simulink model "mu_estimate"  (R2021b)
settings: Solver=ode4  StartTime=0.0  StopTime=5  FixedStep=0.001  RelTol=1e-3
values from neighbouring files (symbols this model uses):
  afx_f = [1.736519934348130,-2.903281841026900e-04,2.651682004580759,7.000047010028531e+04,3.270011055825476e+03,-0.001252141095807,1.596836353939939]    [VehicleParamsFEM20.m]    (also in VehicleParamsFEM20_Gear17.m; VehicleParamsFEM21.m)
  agx_f = [0.230000000000000,2.936116597489246e+04,7.137436879966481e+03,0,0]    [VehicleParamsFEM20.m]    (also in VehicleParamsFEM20_Gear17.m; VehicleParamsFEM21.m)
  Cd = Cd/(40/3.6)^2    (= 0.6885)    [VehicleParamsFEM20.m]    (also in VehicleParamsFEM20_Gear17.m; VehicleParamsFEM21.m)
  Fd = 60*2    (= 120)    [VehicleParamsFEM20.m]    (also in VehicleParamsFEM20_Gear17.m; VehicleParamsFEM21.m)
  g = 9.80665    [VehicleParamsFEM20.m]    (also in VehicleParamsFEM20_Gear17.m; VehicleParamsFEM21.m)
  Iwf = 0.2    [VehicleParamsFEM20.m]    (also in VehicleParamsFEM20_Gear17.m; VehicleParamsFEM21.m)
  Iwr = 0.2    [VehicleParamsFEM20.m]    (also in VehicleParamsFEM20_Gear17.m; VehicleParamsFEM21.m)
  M = 200+60    (= 260)    [VehicleParamsFEM20.m]    (also in VehicleParamsFEM20_Gear17.m; VehicleParamsFEM21.m)
  mu_tire_F = 0.587-0.587+0.55    (= 0.55)    [VehicleParamsFEM20.m]    (also in VehicleParamsFEM20_Gear17.m; VehicleParamsFEM21.m)
  Rwf = 18*(25.4/1000)/2    (= 0.2286)    [VehicleParamsFEM20.m]    (also in VehicleParamsFEM20_Gear17.m; VehicleParamsFEM21.m)
  Rwr = 18*(25.4/1000)/2    (= 0.2286)    [VehicleParamsFEM20.m]    (also in VehicleParamsFEM20_Gear17.m; VehicleParamsFEM21.m)
undefined symbols (not defined in the file or in its folder): mu_diff
libraries: simulink x4, dspstat3 x4
settings Model: Creator=tsuyoshi  LastModifiedBy=tsuyoshi

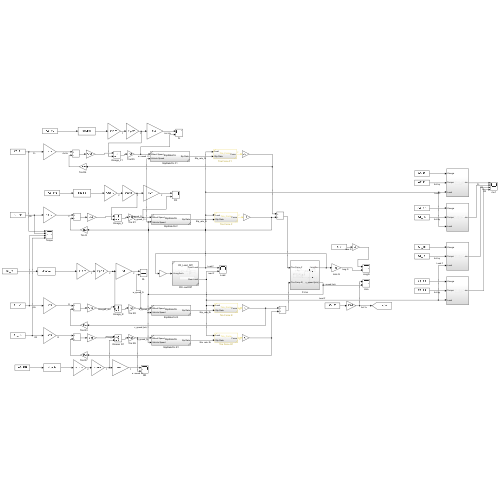
[thumbnail: Simulink's stored preview of the top-level diagram]
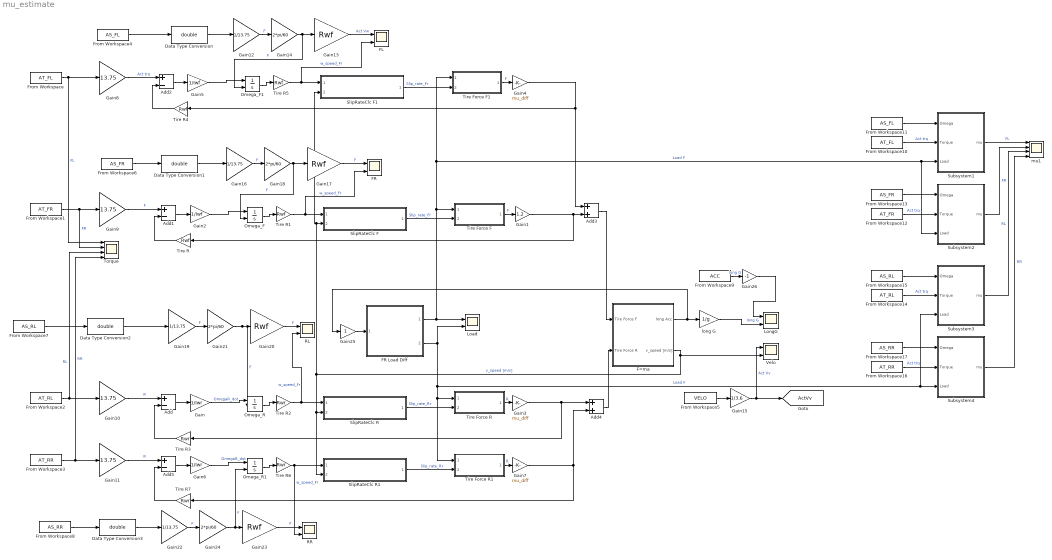
== system mu_estimate ==
  Add{,1..2,5} (4 alike) : Sum  Inputs=+-
  Add3 : Sum
  Add4 : Sum
  Data Type Conversion{,1..3} (4 alike) : DataTypeConversion  OutDataTypeStr=double
  F=ma : Subsystem
  FL : Scope  NumInputPorts=2
  FR : Scope  NumInputPorts=2
  FR Load Diff : Subsystem  ReferencedSubsystem=FR_Load_Diff
  From Workspace : FromWorkspace  VariableName=AT_FL
  From Workspace1 : FromWorkspace  VariableName=AT_FR
  From Workspace10 : FromWorkspace  VariableName=AT_FL
  From Workspace11 : FromWorkspace  VariableName=AS_FL
  From Workspace12 : FromWorkspace  VariableName=AT_FR
  From Workspace13 : FromWorkspace  VariableName=AS_FR
  From Workspace14 : FromWorkspace  VariableName=AT_RL
  From Workspace15 : FromWorkspace  VariableName=AS_RL
  From Workspace16 : FromWorkspace  VariableName=AT_RR
  From Workspace17 : FromWorkspace  VariableName=AS_RR
  From Workspace2 : FromWorkspace  VariableName=AT_RL
  From Workspace3 : FromWorkspace  VariableName=AT_RR
  From Workspace4 : FromWorkspace  VariableName=AS_FL
  From Workspace5 : FromWorkspace  VariableName=VELO
  From Workspace6 : FromWorkspace  VariableName=AS_FR
  From Workspace7 : FromWorkspace  VariableName=AS_RL
  From Workspace8 : FromWorkspace  VariableName=AS_RR
  From Workspace9 : FromWorkspace  VariableName=ACC
  Gain : Gain  Gain=1/Iwr
  Gain1 : Gain  Gain=1.2
  Gain{8..11} (4 alike) : Gain  Gain=13.75
  Gain{12,16,19,22} (4 alike) : Gain  Gain=1/13.75
  Gain{13,17,20,23} (4 alike) : Gain  Gain=Rwf
  Gain{14,18,21,24} (4 alike) : Gain  Gain=2*pi/60
  Gain15 : Gain  Gain=1/3.6
  Gain2 : Gain  Gain=1/Iwf
  Gain25 : Gain
  Gain26 : Gain  Gain=-1
  Gain3 : Gain  Gain=mu_diff
  Gain4 : Gain  Gain=mu_diff
  Gain5 : Gain  Gain=1/Iwf
  Gain6 : Gain  Gain=1/Iwr
  Gain7 : Gain  Gain=mu_diff
  Load : Scope  NumInputPorts=2
  LongG : Scope  NumInputPorts=2
  Omega_F : Integrator  InitialConditionSource=external  LowerSaturationLimit=0
  Omega_F1 : Integrator  InitialConditionSource=external  LowerSaturationLimit=0
  Omega_R : Integrator  InitialConditionSource=external  LowerSaturationLimit=0
  Omega_R1 : Integrator  InitialConditionSource=external  LowerSaturationLimit=0
  RL : Scope  NumInputPorts=2
  RR : Scope  NumInputPorts=2
  SlipRateClc F : Subsystem  ReferencedSubsystem=SlipRateClc
  SlipRateClc F1 : Subsystem  ReferencedSubsystem=SlipRateClc
  SlipRateClc R : Subsystem  ReferencedSubsystem=SlipRateClc
  SlipRateClc R1 : Subsystem  ReferencedSubsystem=SlipRateClc
  Subsystem1 : Subsystem
  Subsystem2 : Subsystem
  Subsystem3 : Subsystem
  Subsystem4 : Subsystem
  Tire Force F : Subsystem  ReferencedSubsystem=Tire_Force
  Tire Force F1 : Subsystem  ReferencedSubsystem=Tire_Force
  Tire Force R : Subsystem  ReferencedSubsystem=Tire_Force
  Tire Force R1 : Subsystem  ReferencedSubsystem=Tire_Force
  Tire R{,1,4..5} (4 alike) : Gain  Gain=Rwf
  Tire R{2..3,6..7} (4 alike) : Gain  Gain=Rwr
  Torque : Scope  NumInputPorts=4
  Velo : Scope  NumInputPorts=2
  long G : Gain  Gain=1/g
  mu1 : Scope  NumInputPorts=4
  tag scope: ActVv=global
  wires:
  Gain3/1 -> Add4/1, Tire R3/1
  SlipRateClc F/1 -> Tire Force F/2  "Slip_rate_Fr"
  Gain1/1 -> Add3/2, Tire R/1
  Add1/1 -> Gain2/1
  Add/1 -> Gain/1
  Gain9/1 -> Add1/1  "F"
  Tire R3/1 -> Add/2
  Add4/1 -> F=ma/2(Tire Force R)
  Tire R/1 -> Add1/2
  Omega_R/1 -> Tire R2/1
  Omega_F/1 -> Tire R1/1
  long G/1 -> LongG/2  "long G"
  Tire Force F/1 -> Gain1/1  "F"
  Gain10/1 -> Add/1  "R"
  Gain2/1 -> Omega_F/1
  F=ma/1(long Acc) -> Gain25/1, long G/1
  Tire Force R/1 -> Gain3/1  "R"
  Gain/1 -> Omega_R/1  "OmegaR_dot"
  SlipRateClc R/1 -> Tire Force R/2  "Slip_rate_Rr"
  Gain5/1 -> Omega_F1/1
  Tire Force F1/1 -> Gain4/1  "F"
  Omega_F1/1 -> Tire R5/1
  Tire R5/1 -> FL/2, SlipRateClc F1/1  "w_speed_Fr"
  Tire R4/1 -> Add2/2
  Gain8/1 -> Add2/1  "Act trq"
  Add2/1 -> Gain5/1
  SlipRateClc F1/1 -> Tire Force F1/2  "Slip_rate_Fr"
  Add3/1 -> F=ma/1(Tire Force F)
  SlipRateClc R1/1 -> Tire Force R1/2  "Slip_rate_Rr"
  Gain6/1 -> Omega_R1/1  "OmegaR_dot"
  Tire Force R1/1 -> Gain7/1  "R"
  F=ma/2(v_speed [m/s]) -> SlipRateClc R1/2, SlipRateClc R/2, SlipRateClc F1/2, SlipRateClc F/2, Velo/2  "v_speed [m/s]"
  Omega_R1/1 -> Tire R6/1
  Tire R7/1 -> Add5/2
  Add5/1 -> Gain6/1
  Gain7/1 -> Tire R7/1, Add4/2
  From Workspace/1 -> Torque/1, Gain8/1  "FL"
  From Workspace1/1 -> Torque/2, Gain9/1  "FR"
  From Workspace2/1 -> Torque/3, Gain10/1  "RL"
  From Workspace3/1 -> Torque/4, Gain11/1  "RR"
  Gain11/1 -> Add5/1  "R"
  From Workspace4/1 -> Data Type Conversion/1
  Gain12/1 -> Gain14/1  "F"
  Gain14/1 -> Omega_F1/2, Gain13/1  "F"
  Gain13/1 -> FL/1  "Act Vw"
  From Workspace5/1 -> Gain15/1
  Gain17/1 -> FR/1  "F"
  Gain18/1 -> Omega_F/2, Gain17/1  "F"
  Gain16/1 -> Gain18/1  "F"
  From Workspace6/1 -> Data Type Conversion1/1
  Tire R1/1 -> FR/2, SlipRateClc F/1  "w_speed_Fr"
  Tire R2/1 -> RL/2, SlipRateClc R/1  "w_speed_Fr"
  Data Type Conversion2/1 -> Gain19/1
  Gain19/1 -> Gain21/1  "F"
  Gain21/1 -> Gain20/1, Omega_R/2  "F"
  Gain20/1 -> RL/1  "F"
  Gain23/1 -> RR/1  "F"
  Gain24/1 -> Omega_R1/2, Gain23/1  "F"
  Gain22/1 -> Gain24/1  "F"
  Data Type Conversion3/1 -> Gain22/1
  Tire R6/1 -> RR/2, SlipRateClc R1/1  "w_speed_Fr"
  Data Type Conversion/1 -> Gain12/1
  Data Type Conversion1/1 -> Gain16/1
  From Workspace7/1 -> Data Type Conversion2/1
  From Workspace8/1 -> Data Type Conversion3/1
  Gain25/1 -> FR Load Diff/1
  From Workspace9/1 -> Gain26/1  "long G"
  Gain26/1 -> LongG/1
  Gain4/1 -> Tire R4/1, Add3/1
  Gain15/1 -> [ActVv], Velo/1  "Act Vv"
  From Workspace11/1 -> Subsystem1/1(Omega)
  From Workspace10/1 -> Subsystem1/2(Torque)  "Act trq"
  Subsystem1/1(mu) -> mu1/1  "FL"
  From Workspace12/1 -> Subsystem2/2(Torque)  "Act trq"
  From Workspace13/1 -> Subsystem2/1(Omega)
  FR Load Diff/1 -> Load/1, Tire Force F1/1, Subsystem2/3(Load), Subsystem1/3(Load), Tire Force F/1  "Load F"
  Subsystem2/1(mu) -> mu1/2  "FR"
  FR Load Diff/2 -> Load/2, Subsystem4/3(Load), Subsystem3/3(Load), Tire Force R1/1, Tire Force R/1  "Load F"
  From Workspace17/1 -> Subsystem4/1(Omega)
  From Workspace16/1 -> Subsystem4/2(Torque)  "Act trq"
  From Workspace14/1 -> Subsystem3/2(Torque)  "Act trq"
  From Workspace15/1 -> Subsystem3/1(Omega)
  Subsystem3/1(mu) -> mu1/3  "RL"
  Subsystem4/1(mu) -> mu1/4  "RR"

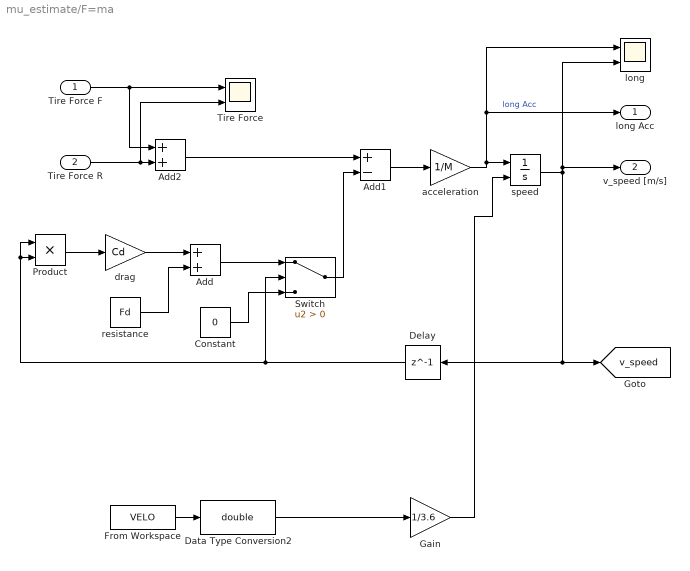
== system mu_estimate/F=ma ==
  Tire Force F : Inport
  Tire Force R : Inport  Port=2
  Add : Sum
  Add1 : Sum  Inputs=+-
  Add2 : Sum
  Constant : Constant  Value=0
  Data Type Conversion2 : DataTypeConversion  OutDataTypeStr=double
  Delay : Delay  DelayLength=1
  From Workspace : FromWorkspace  VariableName=VELO
  Gain : Gain  Gain=1/3.6
  Product : Product
  Switch : Switch  Criteria=u2 > Threshold
  Tire Force : Scope  NumInputPorts=2
  acceleration : Gain  Gain=1/M
  drag : Gain  Gain=Cd
  long : Scope  NumInputPorts=2
  resistance : Constant  Value=Fd
  speed : Integrator  InitialConditionSource=external  LowerSaturationLimit=0
  long Acc : Outport
  v_speed [m/s] : Outport  Port=2
  tag scope: v_speed=global
  wires:
  resistance/1 -> Add/2
  Switch/1 -> Add1/2
  Constant/1 -> Switch/3
  Add1/1 -> acceleration/1
  Add2/1 -> Add1/1
  speed/1 -> long/2, v_speed [m/s]/1, [v_speed], Delay/1
  Add/1 -> Switch/1
  drag/1 -> Add/1
  Product/1 -> drag/1
  Tire Force R/1 -> Tire Force/2, Add2/2
  Tire Force F/1 -> Tire Force/1, Add2/1
  acceleration/1 -> long/1, long Acc/1, speed/1  "long Acc"
  Delay/1 -> Switch/2, Product/1, Product/2
  Data Type Conversion2/1 -> Gain/1
  Gain/1 -> speed/2
  From Workspace/1 -> Data Type Conversion2/1

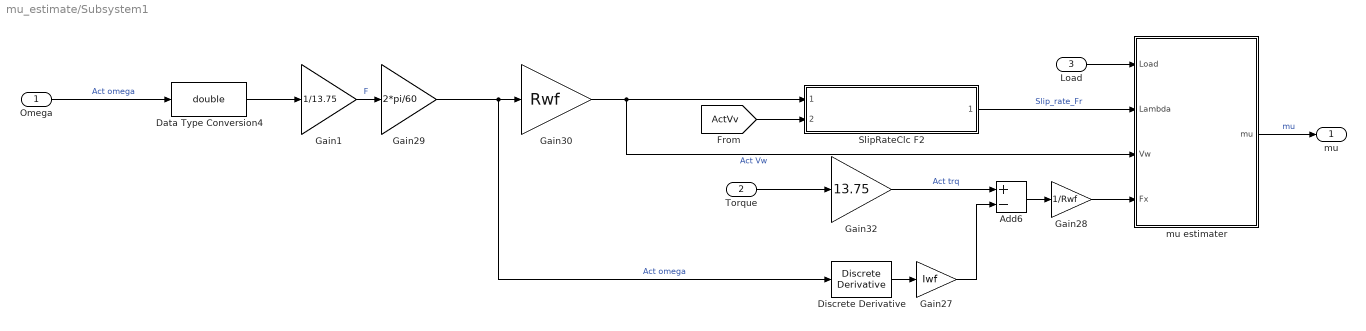
== system mu_estimate/Subsystem1 ==
  Omega : Inport
  Torque : Inport  Port=2
  Load : Inport  Port=3
  Add6 : Sum  Inputs=+-
  Data Type Conversion4 : DataTypeConversion  OutDataTypeStr=double
  Discrete Derivative : simulink/Discrete/Discrete Derivative  gainval=1.0  ICPrevScaledInput=0.0  OutMin=[]  OutMax=[]  OutDataType=fixdt(1, 16)  OutScaling=2^-10  DoSatur=off
  Gain1 : Gain  Gain=1/13.75
  Gain27 : Gain  Gain=Iwf
  Gain28 : Gain  Gain=1/Rwf
  Gain29 : Gain  Gain=2*pi/60
  Gain30 : Gain  Gain=Rwf
  Gain32 : Gain  Gain=13.75
  SlipRateClc F2 : Subsystem  ReferencedSubsystem=SlipRateClc
  mu estimater : Subsystem
  mu : Outport
  wires:
  Add6/1 -> Gain28/1
  Gain30/1 -> mu estimater/3(Vw), SlipRateClc F2/1  "Act Vw"
  Gain29/1 -> Discrete Derivative/1, Gain30/1  "Act omega"
  Load/1 -> mu estimater/1(Load)
  Gain27/1 -> Add6/2
  Gain28/1 -> mu estimater/4(Fx)
  Discrete Derivative/1 -> Gain27/1
  SlipRateClc F2/1 -> mu estimater/2(Lambda)  "Slip_rate_Fr"
  Torque/1 -> Gain32/1
  mu estimater/1(mu) -> mu/1  "mu"
  [ActVv] -> SlipRateClc F2/2
  Gain1/1 -> Gain29/1  "F"
  Data Type Conversion4/1 -> Gain1/1
  Omega/1 -> Data Type Conversion4/1  "Act omega"
  Gain32/1 -> Add6/1  "Act trq"

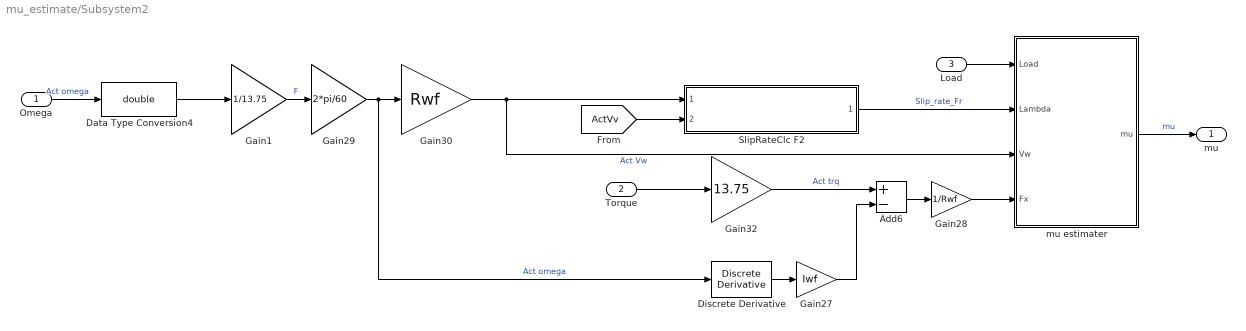
== system mu_estimate/Subsystem2 ==
  Omega : Inport
  Torque : Inport  Port=2
  Load : Inport  Port=3
  Add6 : Sum  Inputs=+-
  Data Type Conversion4 : DataTypeConversion  OutDataTypeStr=double
  Discrete Derivative : simulink/Discrete/Discrete Derivative  gainval=1.0  ICPrevScaledInput=0.0  OutMin=[]  OutMax=[]  OutDataType=fixdt(1, 16)  OutScaling=2^-10  DoSatur=off
  Gain1 : Gain  Gain=1/13.75
  Gain27 : Gain  Gain=Iwf
  Gain28 : Gain  Gain=1/Rwf
  Gain29 : Gain  Gain=2*pi/60
  Gain30 : Gain  Gain=Rwf
  Gain32 : Gain  Gain=13.75
  SlipRateClc F2 : Subsystem  ReferencedSubsystem=SlipRateClc
  mu estimater : Subsystem
  mu : Outport
  wires:
  Gain32/1 -> Add6/1  "Act trq"
  Omega/1 -> Data Type Conversion4/1  "Act omega"
  Data Type Conversion4/1 -> Gain1/1
  Gain1/1 -> Gain29/1  "F"
  [ActVv] -> SlipRateClc F2/2
  mu estimater/1(mu) -> mu/1  "mu"
  Torque/1 -> Gain32/1
  SlipRateClc F2/1 -> mu estimater/2(Lambda)  "Slip_rate_Fr"
  Discrete Derivative/1 -> Gain27/1
  Gain28/1 -> mu estimater/4(Fx)
  Gain27/1 -> Add6/2
  Load/1 -> mu estimater/1(Load)
  Gain29/1 -> Gain30/1, Discrete Derivative/1  "Act omega"
  Gain30/1 -> SlipRateClc F2/1, mu estimater/3(Vw)  "Act Vw"
  Add6/1 -> Gain28/1

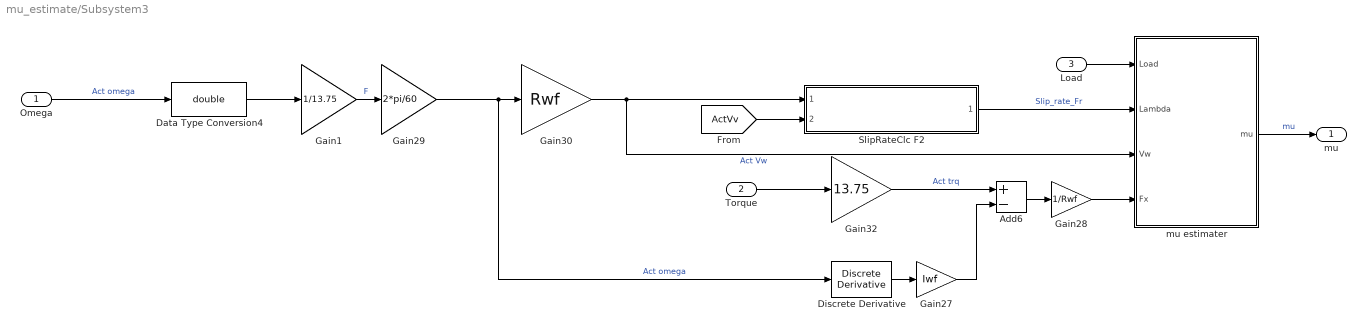
== system mu_estimate/Subsystem3 ==
  Omega : Inport
  Torque : Inport  Port=2
  Load : Inport  Port=3
  Add6 : Sum  Inputs=+-
  Data Type Conversion4 : DataTypeConversion  OutDataTypeStr=double
  Discrete Derivative : simulink/Discrete/Discrete Derivative  gainval=1.0  ICPrevScaledInput=0.0  OutMin=[]  OutMax=[]  OutDataType=fixdt(1, 16)  OutScaling=2^-10  DoSatur=off
  Gain1 : Gain  Gain=1/13.75
  Gain27 : Gain  Gain=Iwf
  Gain28 : Gain  Gain=1/Rwf
  Gain29 : Gain  Gain=2*pi/60
  Gain30 : Gain  Gain=Rwf
  Gain32 : Gain  Gain=13.75
  SlipRateClc F2 : Subsystem  ReferencedSubsystem=SlipRateClc
  mu estimater : Subsystem
  mu : Outport
  wires:
  Add6/1 -> Gain28/1
  Gain30/1 -> mu estimater/3(Vw), SlipRateClc F2/1  "Act Vw"
  Gain29/1 -> Discrete Derivative/1, Gain30/1  "Act omega"
  Load/1 -> mu estimater/1(Load)
  Gain27/1 -> Add6/2
  Gain28/1 -> mu estimater/4(Fx)
  Discrete Derivative/1 -> Gain27/1
  SlipRateClc F2/1 -> mu estimater/2(Lambda)  "Slip_rate_Fr"
  Torque/1 -> Gain32/1
  mu estimater/1(mu) -> mu/1  "mu"
  [ActVv] -> SlipRateClc F2/2
  Gain1/1 -> Gain29/1  "F"
  Data Type Conversion4/1 -> Gain1/1
  Omega/1 -> Data Type Conversion4/1  "Act omega"
  Gain32/1 -> Add6/1  "Act trq"

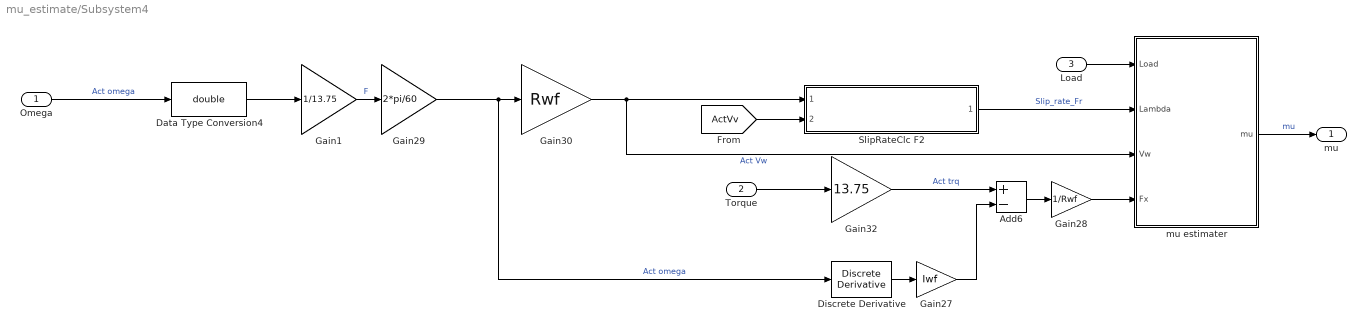
== system mu_estimate/Subsystem4 ==
  Omega : Inport
  Torque : Inport  Port=2
  Load : Inport  Port=3
  Add6 : Sum  Inputs=+-
  Data Type Conversion4 : DataTypeConversion  OutDataTypeStr=double
  Discrete Derivative : simulink/Discrete/Discrete Derivative  gainval=1.0  ICPrevScaledInput=0.0  OutMin=[]  OutMax=[]  OutDataType=fixdt(1, 16)  OutScaling=2^-10  DoSatur=off
  Gain1 : Gain  Gain=1/13.75
  Gain27 : Gain  Gain=Iwf
  Gain28 : Gain  Gain=1/Rwf
  Gain29 : Gain  Gain=2*pi/60
  Gain30 : Gain  Gain=Rwf
  Gain32 : Gain  Gain=13.75
  SlipRateClc F2 : Subsystem  ReferencedSubsystem=SlipRateClc
  mu estimater : Subsystem
  mu : Outport
  wires:
  Gain32/1 -> Add6/1  "Act trq"
  Omega/1 -> Data Type Conversion4/1  "Act omega"
  Data Type Conversion4/1 -> Gain1/1
  Gain1/1 -> Gain29/1  "F"
  [ActVv] -> SlipRateClc F2/2
  mu estimater/1(mu) -> mu/1  "mu"
  Torque/1 -> Gain32/1
  SlipRateClc F2/1 -> mu estimater/2(Lambda)  "Slip_rate_Fr"
  Discrete Derivative/1 -> Gain27/1
  Gain28/1 -> mu estimater/4(Fx)
  Gain27/1 -> Add6/2
  Load/1 -> mu estimater/1(Load)
  Gain29/1 -> Gain30/1, Discrete Derivative/1  "Act omega"
  Gain30/1 -> SlipRateClc F2/1, mu estimater/3(Vw)  "Act Vw"
  Add6/1 -> Gain28/1

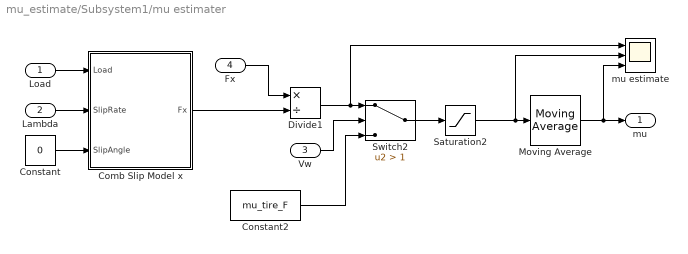
== system mu_estimate/Subsystem1/mu estimater ==
  Load : Inport
  Lambda : Inport  Port=2
  Vw : Inport  Port=3
  Fx : Inport  Port=4
  Comb Slip Model x : MATLAB Function  TreatAsAtomicUnit=on
  Constant : Constant  Value=0
  Constant2 : Constant  Value=mu_tire_F
  Divide1 : Product  Inputs=*/
  Moving Average : dspstat3/Moving Average  Method=Sliding window  ForgettingFactorPort=off  SpecifyWindowLength=on  WindowLength=50  ForgettingFactor=0.9  SimulateUsing=Code generation
  Saturation2 : Saturate  UpperLimit=1  LowerLimit=0
  Switch2 : Switch  Criteria=u2 > Threshold  Threshold=1
  mu estimate : Scope  NumInputPorts=3
  mu : Outport
  wires:
  Constant2/1 -> Switch2/3
  Saturation2/1 -> mu estimate/2, Moving Average/1
  Fx/1 -> Divide1/1
  Moving Average/1 -> mu estimate/3, mu/1
  Divide1/1 -> mu estimate/1, Switch2/1
  Vw/1 -> Switch2/2
  Switch2/1 -> Saturation2/1
  Comb Slip Model x/1(Fx) -> Divide1/2
  Load/1 -> Comb Slip Model x/1(Load)
  Lambda/1 -> Comb Slip Model x/2(SlipRate)
  Constant/1 -> Comb Slip Model x/3(SlipAngle)

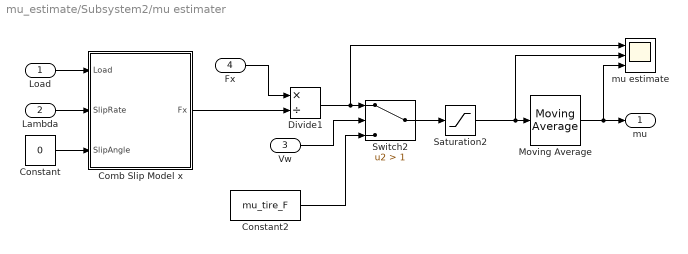
== system mu_estimate/Subsystem2/mu estimater ==
  Load : Inport
  Lambda : Inport  Port=2
  Vw : Inport  Port=3
  Fx : Inport  Port=4
  Comb Slip Model x : MATLAB Function  TreatAsAtomicUnit=on
  Constant : Constant  Value=0
  Constant2 : Constant  Value=mu_tire_F
  Divide1 : Product  Inputs=*/
  Moving Average : dspstat3/Moving Average  Method=Sliding window  ForgettingFactorPort=off  SpecifyWindowLength=on  WindowLength=50  ForgettingFactor=0.9  SimulateUsing=Code generation
  Saturation2 : Saturate  UpperLimit=1  LowerLimit=0
  Switch2 : Switch  Criteria=u2 > Threshold  Threshold=1
  mu estimate : Scope  NumInputPorts=3
  mu : Outport
  wires:
  Constant/1 -> Comb Slip Model x/3(SlipAngle)
  Lambda/1 -> Comb Slip Model x/2(SlipRate)
  Load/1 -> Comb Slip Model x/1(Load)
  Comb Slip Model x/1(Fx) -> Divide1/2
  Switch2/1 -> Saturation2/1
  Vw/1 -> Switch2/2
  Divide1/1 -> Switch2/1, mu estimate/1
  Moving Average/1 -> mu/1, mu estimate/3
  Fx/1 -> Divide1/1
  Saturation2/1 -> Moving Average/1, mu estimate/2
  Constant2/1 -> Switch2/3

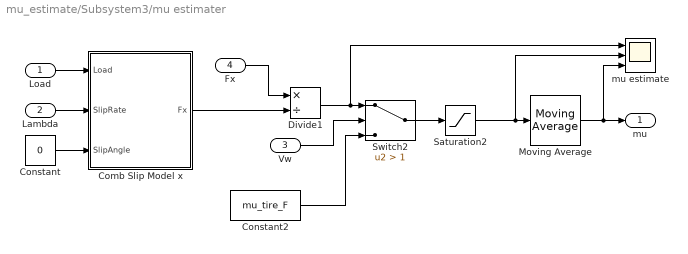
== system mu_estimate/Subsystem3/mu estimater ==
  Load : Inport
  Lambda : Inport  Port=2
  Vw : Inport  Port=3
  Fx : Inport  Port=4
  Comb Slip Model x : MATLAB Function  TreatAsAtomicUnit=on
  Constant : Constant  Value=0
  Constant2 : Constant  Value=mu_tire_F
  Divide1 : Product  Inputs=*/
  Moving Average : dspstat3/Moving Average  Method=Sliding window  ForgettingFactorPort=off  SpecifyWindowLength=on  WindowLength=50  ForgettingFactor=0.9  SimulateUsing=Code generation
  Saturation2 : Saturate  UpperLimit=1  LowerLimit=0
  Switch2 : Switch  Criteria=u2 > Threshold  Threshold=1
  mu estimate : Scope  NumInputPorts=3
  mu : Outport
  wires:
  Constant2/1 -> Switch2/3
  Saturation2/1 -> mu estimate/2, Moving Average/1
  Fx/1 -> Divide1/1
  Moving Average/1 -> mu estimate/3, mu/1
  Divide1/1 -> mu estimate/1, Switch2/1
  Vw/1 -> Switch2/2
  Switch2/1 -> Saturation2/1
  Comb Slip Model x/1(Fx) -> Divide1/2
  Load/1 -> Comb Slip Model x/1(Load)
  Lambda/1 -> Comb Slip Model x/2(SlipRate)
  Constant/1 -> Comb Slip Model x/3(SlipAngle)

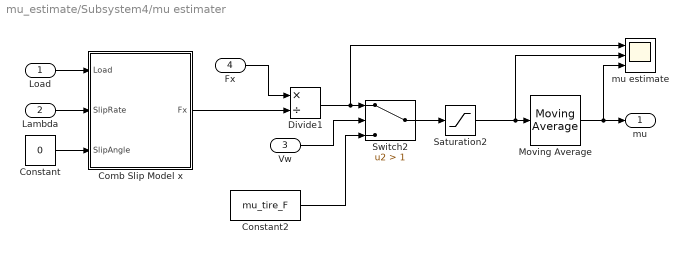
== system mu_estimate/Subsystem4/mu estimater ==
  Load : Inport
  Lambda : Inport  Port=2
  Vw : Inport  Port=3
  Fx : Inport  Port=4
  Comb Slip Model x : MATLAB Function  TreatAsAtomicUnit=on
  Constant : Constant  Value=0
  Constant2 : Constant  Value=mu_tire_F
  Divide1 : Product  Inputs=*/
  Moving Average : dspstat3/Moving Average  Method=Sliding window  ForgettingFactorPort=off  SpecifyWindowLength=on  WindowLength=50  ForgettingFactor=0.9  SimulateUsing=Code generation
  Saturation2 : Saturate  UpperLimit=1  LowerLimit=0
  Switch2 : Switch  Criteria=u2 > Threshold  Threshold=1
  mu estimate : Scope  NumInputPorts=3
  mu : Outport
  wires:
  Constant/1 -> Comb Slip Model x/3(SlipAngle)
  Lambda/1 -> Comb Slip Model x/2(SlipRate)
  Load/1 -> Comb Slip Model x/1(Load)
  Comb Slip Model x/1(Fx) -> Divide1/2
  Switch2/1 -> Saturation2/1
  Vw/1 -> Switch2/2
  Divide1/1 -> Switch2/1, mu estimate/1
  Moving Average/1 -> mu/1, mu estimate/3
  Fx/1 -> Divide1/1
  Saturation2/1 -> Moving Average/1, mu estimate/2
  Constant2/1 -> Switch2/3

== matlab function mu_estimate/Subsystem1/mu estimater/Comb Slip Model x ==
  data: Load input; SlipRate input; Fx output; SlipAngle input; agx_f parameter; afx_f parameter
function Fx = fcn(Load, SlipRate, SlipAngle, agx_f, afx_f)
    if Load==0
        Fx=0;
    else
        C = agx_f(1);
        D = fcnPureFx(Load, SlipRate, afx_f);
        E = Load*agx_f(4) + agx_f(5);
        B = agx_f(2)*sin(2*atan(Load/agx_f(3)))/(D*C);
        Fx = D*cos(C*atan(B*SlipAngle-E*(B*SlipAngle-atan(B*SlipAngle))));
    end
end

function PureFx = fcnPureFx(Load, SlipRate, afx_f)
    C = afx_f(1);
    D = (Load*afx_f(2) + afx_f(3))*Load;
    E = Load*afx_f(6) + afx_f(7);
    B = afx_f(4)*sin(2*atan(Load/afx_f(5)))/(D*C);
    PureFx = D*sin(C*atan(B*SlipRate-E*(B*SlipRate-atan(B*SlipRate))));
end

== matlab function mu_estimate/Subsystem2/mu estimater/Comb Slip Model x ==
  data: Load input; SlipRate input; Fx output; SlipAngle input; agx_f parameter; afx_f parameter
function Fx = fcn(Load, SlipRate, SlipAngle, agx_f, afx_f)
    if Load==0
        Fx=0;
    else
        C = agx_f(1);
        D = fcnPureFx(Load, SlipRate, afx_f);
        E = Load*agx_f(4) + agx_f(5);
        B = agx_f(2)*sin(2*atan(Load/agx_f(3)))/(D*C);
        Fx = D*cos(C*atan(B*SlipAngle-E*(B*SlipAngle-atan(B*SlipAngle))));
    end
end

function PureFx = fcnPureFx(Load, SlipRate, afx_f)
    C = afx_f(1);
    D = (Load*afx_f(2) + afx_f(3))*Load;
    E = Load*afx_f(6) + afx_f(7);
    B = afx_f(4)*sin(2*atan(Load/afx_f(5)))/(D*C);
    PureFx = D*sin(C*atan(B*SlipRate-E*(B*SlipRate-atan(B*SlipRate))));
end

== matlab function mu_estimate/Subsystem3/mu estimater/Comb Slip Model x ==
  data: Load input; SlipRate input; Fx output; SlipAngle input; agx_f parameter; afx_f parameter
function Fx = fcn(Load, SlipRate, SlipAngle, agx_f, afx_f)
    if Load==0
        Fx=0;
    else
        C = agx_f(1);
        D = fcnPureFx(Load, SlipRate, afx_f);
        E = Load*agx_f(4) + agx_f(5);
        B = agx_f(2)*sin(2*atan(Load/agx_f(3)))/(D*C);
        Fx = D*cos(C*atan(B*SlipAngle-E*(B*SlipAngle-atan(B*SlipAngle))));
    end
end

function PureFx = fcnPureFx(Load, SlipRate, afx_f)
    C = afx_f(1);
    D = (Load*afx_f(2) + afx_f(3))*Load;
    E = Load*afx_f(6) + afx_f(7);
    B = afx_f(4)*sin(2*atan(Load/afx_f(5)))/(D*C);
    PureFx = D*sin(C*atan(B*SlipRate-E*(B*SlipRate-atan(B*SlipRate))));
end

== matlab function mu_estimate/Subsystem4/mu estimater/Comb Slip Model x ==
  data: Load input; SlipRate input; Fx output; SlipAngle input; agx_f parameter; afx_f parameter
function Fx = fcn(Load, SlipRate, SlipAngle, agx_f, afx_f)
    if Load==0
        Fx=0;
    else
        C = agx_f(1);
        D = fcnPureFx(Load, SlipRate, afx_f);
        E = Load*agx_f(4) + agx_f(5);
        B = agx_f(2)*sin(2*atan(Load/agx_f(3)))/(D*C);
        Fx = D*cos(C*atan(B*SlipAngle-E*(B*SlipAngle-atan(B*SlipAngle))));
    end
end

function PureFx = fcnPureFx(Load, SlipRate, afx_f)
    C = afx_f(1);
    D = (Load*afx_f(2) + afx_f(3))*Load;
    E = Load*afx_f(6) + afx_f(7);
    B = afx_f(4)*sin(2*atan(Load/afx_f(5)))/(D*C);
    PureFx = D*sin(C*atan(B*SlipRate-E*(B*SlipRate-atan(B*SlipRate))));
end
